simulink model "RocketPlant"  (R2024b)
settings: Solver=FixedStepAuto  StartTime=0.0  StopTime=300  FixedStep=.001  RelTol=1e-3
libraries: simulink x1
settings Model: PacingRate=0.630000  Creator=xavie  LastModifiedBy=olive
settings DataIOCC: LoggingFileName=rocket.mat
settings RTWCC: GPUComputeCapability=3.5

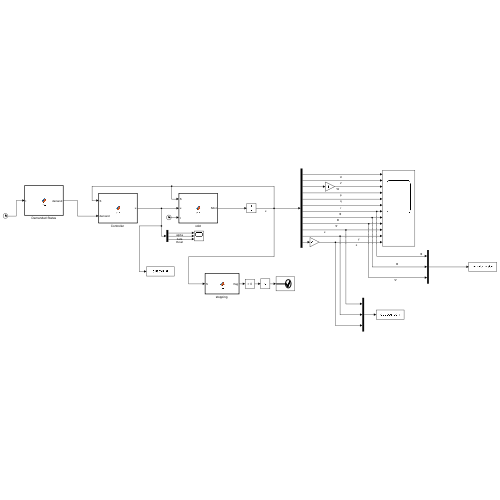
[thumbnail: Simulink's stored preview of the top-level diagram]
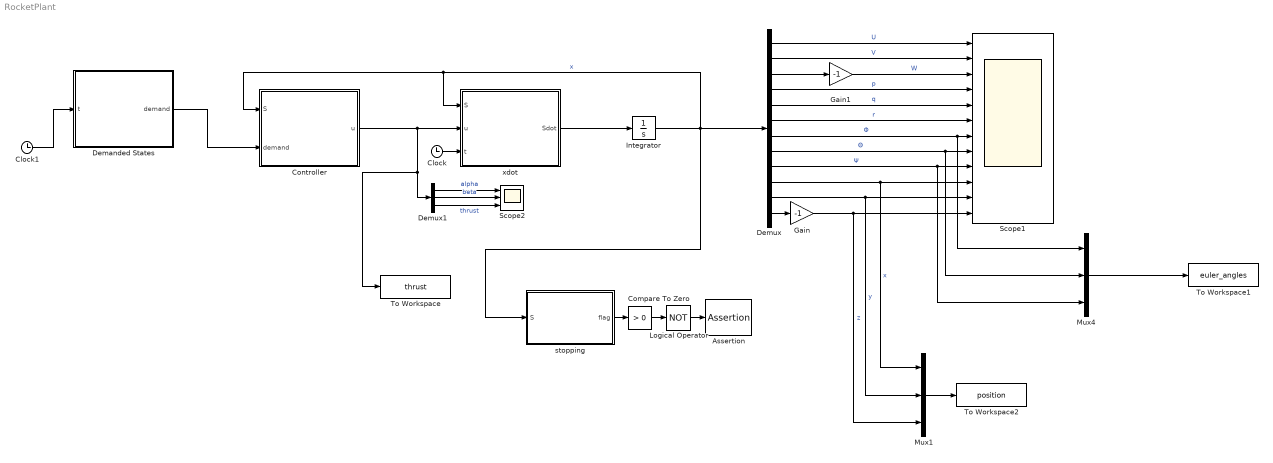
== system RocketPlant ==
  Assertion : Assertion
  Clock : Clock
  Clock1 : Clock
  Compare To Zero : simulink/Logic and Bit Operations/Compare To Zero  relop=>  OutDataTypeStr=boolean
  "Controller " : MATLAB Function  TreatAsAtomicUnit=on
  Demanded States : MATLAB Function  TreatAsAtomicUnit=on
  Demux : Demux  Outputs=12
  Demux1 : Demux  Outputs=3
  Gain : Gain  Gain=-1
  Gain1 : Gain  Gain=-1
  Integrator : Integrator  InitialCondition=[0;0;0;0;0;0;0;0;0;0;0;0]
  Logical Operator : Logic  Operator=NOT  AllPortsSameDT=off  OutDataTypeStr=boolean
  Mux1 : Mux  Inputs=3
  Mux4 : Mux  Inputs=3
  Scope1 : Scope  NumInputPorts=12
  Scope2 : Scope  NumInputPorts=3
  To Workspace : ToWorkspace  VariableName=thrust  SaveFormat=Timeseries  SampleTime=-1
  To Workspace1 : ToWorkspace  VariableName=euler_angles  SaveFormat=Timeseries  SampleTime=-1
  To Workspace2 : ToWorkspace  VariableName=position  SaveFormat=Timeseries  SampleTime=-1
  "stopping " : MATLAB Function  TreatAsAtomicUnit=on
  xdot : MATLAB Function  TreatAsAtomicUnit=on
  wires:
  xdot/1(Sdot) -> Integrator/1
  Integrator/1 -> "stopping "/1(S), Demux/1, xdot/1(S), "Controller "/1(S)  "x"
  "Controller "/1(u) -> To Workspace/1, Demux1/1, xdot/2(u)
  Demux/1 -> Scope1/1  "U"
  Demux/2 -> Scope1/2  "V"
  Demux/3 -> Gain1/1
  Demux/4 -> Scope1/4  "p"
  Demux/5 -> Scope1/5  "q"
  Demux/6 -> Scope1/6  "r"
  Demux/10 -> Scope1/10, Mux1/1  "x"
  Demux/11 -> Mux1/2, Scope1/11  "y"
  Demux/12 -> Gain/1
  Clock/1 -> xdot/3(t)
  Demux1/1 -> Scope2/1  "alpha"
  Demux1/2 -> Scope2/2  "beta"
  Demux1/3 -> Scope2/3  "thrust"
  "stopping "/1(flag) -> Compare To Zero/1
  Compare To Zero/1 -> Logical Operator/1
  Logical Operator/1 -> Assertion/1
  Gain/1 -> Mux1/3, Scope1/12  "z"
  Gain1/1 -> Scope1/3  "W"
  Clock1/1 -> Demanded States/1(t)
  Demanded States/1(demand) -> "Controller "/2(demand)
  Mux4/1 -> To Workspace1/1
  Demux/7 -> Mux4/1, Scope1/7  "Φ"
  Demux/8 -> Mux4/2, Scope1/8  "Θ"
  Demux/9 -> Mux4/3, Scope1/9  "Ψ"
  Mux1/1 -> To Workspace2/1

== matlab function RocketPlant/Controller  ==
  settings: updateMethod=DISCRETE
  data: S input; u output; demand input
function u = fcn(S,demand)
%{
Takes in thrust, angles of thrust, x and outputs xdot
Body axis is defined as z being the in the direction of gravity when pitch
is zero
mass-kg
I - moment of inertia - kg m^2
cg - centre of gravity - m
thrust position - m
p:


x: 
U - body axis x velocity - m/s
V - body axis y velocity - m/s
W - body axis z velocity - m/s
p - body axis roll rate - rad/s
q - body axis pitch rate - rad/s
r - body axis yaw rate - rad/s
phi - earth axis roll - rad
theta - earth axis pitch - rad
psi - earth axis yaw - rad

u: 
alpha - Gimbal angle 1
beta - Gimbal angle 2
T - Thrust  
%}


    %% Extract state variables
    U = S(1);
    V = S(2); 
    W = S(3);
    p = S(4);
    q = S(5); 
    r = S(6);
    phi = S(7); 
    theta = S(8); 
    psi = S(9);
    x = S(10); 
    y = S(11); 
    z = S(12);

    %% Desired target positions (demands)
    dem_x = 0; % Target x position (m)
    dem_y = 0; % Target y position (m)
    dem_z = 0; % Target z position (m)
    dem_phi = demand(4); % target angle phi (rad)
    dem_theta = demand(5);% target angle theta (rad)
    
    %% PID gains
    % Gimbal angle 1 (alpha) control gains
    Kp_a = 5; Ki_a = 0; Kd_a = 1000;

    % Gimbal angle 2 (beta) control gains
    Kp_b =5; Ki_b = 0; Kd_b = 1000;
    % Kp_b =0; Ki_b = 0.00000; Kd_b = 000;
    
    % Thrust (T) control gains
    Kp_t =7; Ki_t = 0.00015; Kd_t = 42000;
    
    %% Persistent variables for PID state
    % Integral terms for continuous accumulation
    persistent integral_x integral_y integral_z integral_phi integral_theta;
    % Derivative terms for tracking previous errors
    persistent prev_error_x prev_error_y prev_error_z prev_error_phi prev_error_theta;

    % Initialize persistent variables if this is the first call
    if isempty(integral_x)
        integral_x = 0; 
        integral_y = 0; 
        integral_z = 0;
        integral_phi = 0;
        integral_theta = 0;

        prev_error_x = 0; 
        prev_error_y = 0; 
        prev_error_z = 0;
        prev_error_phi = 0;
        prev_error_theta = 0;
    end

    %% Compute errors
    % Positional errors in x, y, and z
    error_x = dem_x - x;
    error_y = dem_y - y;
    error_z = dem_z - z;

    error_phi = dem_phi - phi;
    error_theta = dem_theta - theta;

    %% Update integral terms (continuous accumulation of error)
    % Integrators accumulate error over time naturally in continuous time
    integral_x = integral_x + error_x;
    integral_y = integral_y + error_y;
    integral_z = integral_z + error_z;

    integral_phi = integral_phi + error_phi;
    integral_theta = integral_theta + error_theta;

    %% Compute derivative terms (rate of change of error)
    % In continuous time, these represent the instantaneous rate of error change
    derivative_x = error_x - prev_error_x;
    derivative_y = error_y - prev_error_y;
    derivative_z = error_z - prev_error_z;
    
    derivative_phi = error_phi - prev_error_phi;
    derivative_theta = error_theta - prev_error_theta;
    %% Compute PID control outputs
    % Gimbal angle 1 (alpha)

        % Calculating using x error
        % u1 = Kp_a * error_x + Ki_a * integral_x + Kd_a * derivative_x;
        % u1=min(max(u1,-pi/12),pi/12);
        
        % Calculating using theta error
        u1 = -1*(Kp_a * error_theta + Ki_a * integral_theta + Kd_a * derivative_theta);
        u1=min(max(u1,-pi/12),pi/12);
    % Gimbal angle 2 (beta)

        % Calculating using y error
        % u2 = Kp_y * error_y + Ki_y * integral_y + Kd_y * derivative_y;
        % u2=min(max(u2,-pi/18),pi/18);

        % calculating using phi error        
        u2=Kp_b * error_phi + Ki_b * integral_phi + Kd_b * derivative_phi;
        u2=min(max(u2,-pi/12),pi/12);

    % Thrust

        % % Thrust Control
        % u3 = -Kp_z * error_z + -Ki_z * integral_z + -Kd_z * derivative_z;
        % u3 = min(max(u3,0),6000);

        % Constant Thrust
        u3 = 1000;

   
    %% Update previous errors for derivative calculation
    prev_error_x = error_x;
    prev_error_y = error_y;
    prev_error_z = error_z;
    prev_error_phi = error_phi;
    prev_error_theta = error_theta;

    %% Combine control outputs into a single vector
    u = [u1; u2; u3];
end

== matlab function RocketPlant/xdot ==
  data: S input; u input; Sdot output; t input
function Sdot = fcn(S, u, t)
 
%Parameters
m=75;
cg=[0,0,units(-2500,'mm','m')];
thrust_pos=[units(0,'mm','m'),units(0,'mm','m'),units(0,'mm','m')];

%%Control input
alpha=u(1); 
beta=u(2);
T=u(3);

%%states
U=S(1);
V=S(2);
W=S(3);
p=S(4);
q=S(5);
r=S(6);
phi=S(7);
theta=S(8);
psi=S(9);
x=S(10);
y=S(11);
z=S(12);

% bounding 
% phi = mod(phi + pi, 2 * pi) - pi;
% theta = mod(theta + pi, 2 * pi) - pi;
% psi = mod(psi + pi, 2 * pi) - pi;
%%Constants


T_etob=[cos(theta)*cos(psi), sin(theta)*sin(phi)*cos(psi)-cos(phi)*sin(psi), cos(phi)*sin(theta)*cos(psi)+sin(phi)*sin(psi);
    cos(theta)*sin(psi), sin(phi)*sin(theta)*sin(psi)+cos(phi)*cos(psi), cos(phi)*sin(theta)*cos(psi)-sin(phi)*cos(psi);
    -sin(theta),sin(phi)*cos(theta), cos(phi)*cos(theta)]';
gb=9.81;
ge=T_etob*[0;0;gb];
gx=ge(1);
gy=ge(2);
gz=ge(3);

% Forces
%alpha is about y and beta is about x
Tx=-T*sin(alpha);
Ty=-T*cos(alpha)*sin(beta); 
Tz=-T*cos(alpha)*cos(beta);

Fx=Tx+m*gx;
Fy=Ty+m*gy;
Fz=Tz+m*gz;

%Compute xdot
Udot=Fx/m-(W*q-V*r);
Vdot=Fy/m-(U*r-p*W);
Wdot=Fz/m-(V*p-U*q);

%%Rotational moments
lx=thrust_pos(1)-cg(1);
ly=thrust_pos(2)-cg(2);
lz=thrust_pos(3)-cg(3);

L=ly*Tz-lz*Ty;
M=-lx*Tz+lz*Tx;
N=lx*Ty-ly*Tx;

%%Mass and inertia

Ixx=79;
Iyy=79;
Izz=0.42;

pdot=(L-q*r*(Izz-Iyy))/Ixx;
qdot=(M-r*p*(Ixx-Izz))/Iyy;
rdot=(N-p*q*(Iyy-Ixx))/Izz;

% Compute Euler angles
AngleCon_btoe=[1, sin(phi)*tan(theta), cos(phi)*tan(theta);
                0, cos(phi), -sin(phi);
                0, sin(phi)*sec(theta), cos(phi)*sec(theta)];
EulerAngledot=AngleCon_btoe*[p;q;r];

% Veclocity
velocity=T_etob\[S(1);S(2);S(3)];

%Compute Xdot
Sdot=[Udot;Vdot;Wdot;pdot;qdot;rdot;EulerAngledot;velocity];

== matlab function RocketPlant/stopping  ==
  data: S input; flag output
function flag = fcn(S)
 if S(12)>0
     flag = 1;
 else flag = 0;
 end
end

== matlab function RocketPlant/Demanded States ==
  settings: updateMethod=DISCRETE
  data: demand output; t input
function demand = fcn(t)

% Define the two different sets of values
if mod(t, 10) < 5
    % First set of values for the first 5 iterations
    dem_x = 0;
    dem_y = 0;
    dem_z = 0;
    dem_phi = 0.2;
    dem_theta = 0.2;
else
    % Second set of values for the next 5 iterations
    dem_x = 0;
    dem_y = 0;
    dem_z = 0;
    dem_phi = -0.2;
    dem_theta = -0.2;
end

% Combine the values into the demand vector
demand = [dem_x; dem_y; dem_z; dem_phi; dem_theta];

end
